simulink model "input_encoder"  (R2019a)
settings: Solver=ode8  StartTime=0.0  StopTime=10.0  FixedStep=0.01  RelTol=1e-3
values from neighbouring files (symbols this model uses):
  input_enc_diff = (input_enc_max - input_enc_min)    (= 196)    [input_encoder_params.m]
  input_enc_diff_thr = input_enc_diff * 0.9    (= 176.4)    [input_encoder_params.m]
undefined symbols (not defined in the file or in its folder): sigbuilder_block
libraries: simulink x3
settings Model: Creator=piotr  LastModifiedBy=piotr

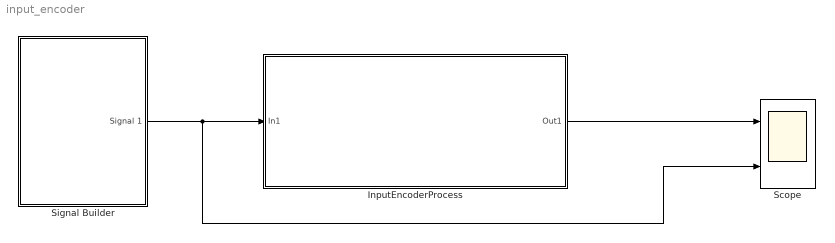
== system input_encoder ==
  InputEncoderProcess : Subsystem
  Scope : Scope  NumInputPorts=2
  Signal Builder : Subsystem  Tag=STV Subsys  LoadFcn=sigbuilder_block('load',[1510.48 257.684 543.411 405.474 ]);  StartFcn=sigbuilder_block('start');  StopFcn=sigbuilder_block('stop');  ClipboardFcn=sigbuilder_block('clipboard');  mask(Sigbuilder block){tuvar=[0:10]}
      mask help: Simulink:masks:SigbuilderBlock_MD
      mask init:
      | if ~strcmp(get_param(bdroot(gcbh),'SimulationStatus'),'stopped') tuvar = sigbuilder_block('maskInit'); end
      settings: CopyFcn=sigbuilder_block('copy');  DeleteFcn=sigbuilder_block('delete');  ModelCloseFcn=sigbuilder_block('modelClose');  PreSaveFcn=sigbuilder_block('preSave');  PauseFcn=sigbuilder_block('pause');  ContinueFcn=sigbuilder_block('continue');  NameChangeFcn=sigbuilder_block('namechange');  OpenFcn=sigbuilder_block('open',[437.6 199.2 550.4 400 ]);  CloseFcn=sigbuilder_block('close');
      mask Display: plot(0, 0, 100, 100,[2, 2, 32, 32, 2], [68, 8, 8, 68, 68],[32, 2], [38, 38], [32, 19, 2],[53, 60, 44], [32, 17, 17, 2],[16, 16, 31, 31]);txt = getActiveGroup(gcbh);text(2, 100, txt,'verticalAlignment', 'top');
  wires:
  Signal Builder/1(Signal 1) -> Scope/2, InputEncoderProcess/1(In1)
  InputEncoderProcess/1(Out1) -> Scope/1

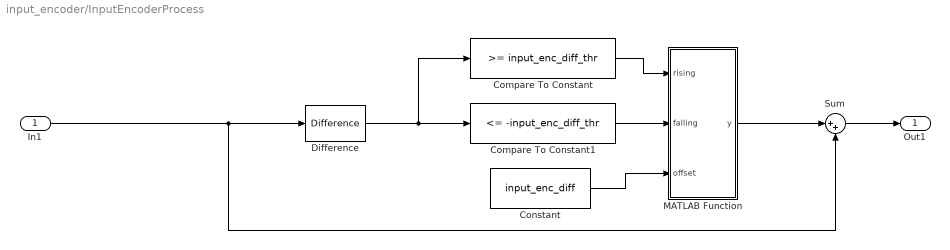
== system input_encoder/InputEncoderProcess ==
  In1 : Inport
  Compare To Constant : simulink/Logic and Bit Operations/Compare To Constant  relop=>=  const=input_enc_diff_thr  OutDataTypeStr=boolean
  Compare To Constant1 : simulink/Logic and Bit Operations/Compare To Constant  relop=<=  const=-input_enc_diff_thr  OutDataTypeStr=boolean
  Constant : Constant  Value=input_enc_diff
  Difference : simulink/Discrete/Difference  ICPrevInput=0.0  OutMin=[]  OutMax=[]  OutDataType=fixdt(1, 16)  OutScaling=2^-10  DoSatur=off
  MATLAB Function : MATLAB Function  TreatAsAtomicUnit=on
  Sum : Sum  Inputs=|++
  Out1 : Outport
  wires:
  Sum/1 -> Out1/1
  In1/1 -> Sum/2, Difference/1
  Difference/1 -> Compare To Constant/1, Compare To Constant1/1
  Compare To Constant1/1 -> MATLAB Function/2(falling)
  Compare To Constant/1 -> MATLAB Function/1(rising)
  Constant/1 -> MATLAB Function/3(offset)
  MATLAB Function/1(y) -> Sum/1

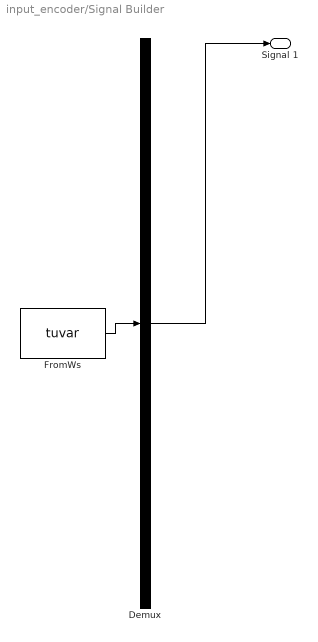
== system input_encoder/Signal Builder ==
  Demux : Demux  Tag=STV Demux  Outputs=1
  FromWs : FromWorkspace  Tag=STV FromWs  VariableName=tuvar  SampleTime=0
      SigBuilderData=|
      | common.afterFinalStr = 'Extrapolate'
      | common.sampleTime = 0
      | dataSet.timeRange = [0 10]
      | dataSet.name = 'Group 1'
      | sbobj.Groups.Name = 'Group 1'
      | sbobj.Groups.Signals.Name = 'Signal 1'
      | sbobj.Groups.Signals.XData = [0 1.34 1.34 2.58 2.58 4.16 4.16 6 6 7.32 7.32 8.68 8.68 10]
      | sbobj.Groups.Signals.YData = [0 0 -97 101 -99 97 -95 105 89 -93 102 -99 0 0]
  Signal 1 : Outport  Tag=STV Outport
  wires:
  Demux/1 -> Signal 1/1
  FromWs/1 -> Demux/1

== matlab function input_encoder/InputEncoderProcess/MATLAB Function ==
  data: rising input; y output; falling input; offset input
function y = fcn(rising, falling, offset)
persistent acc
if isempty(acc)
    acc = 0;
end
if rising == true
    acc = acc - offset;
end
if falling == true
    acc = acc + offset;
end
y = acc;
